simulink model "Reshape_TestGen24"  (R2017b)
settings: Solver=FixedStepDiscrete  StartTime=0.0  StopTime=10.0  RelTol=1e-3
undefined symbols (not defined in the file): Block_TestLib, enable
settings Model: Creator=ktrinh  LastModifiedBy=ktrinh
settings DebuggingCC: ParameterOverflowMsg=none

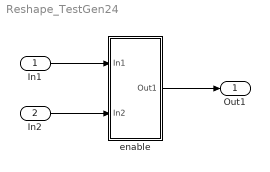
== system Reshape_TestGen24 ==
  In1 : Inport
  In2 : Inport  Port=2
  enable : Subsystem  AncestorBlock=Block_TestLib/enable
  Out1 : Outport
  wires:
  In1/1 -> enable/1(In1)
  In2/1 -> enable/2(In2)
  enable/1(Out1) -> Out1/1

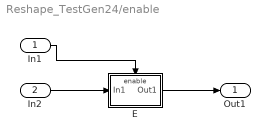
== system Reshape_TestGen24/enable ==
  In1 : Inport  OutDataTypeStr=boolean
  In2 : Inport  Port=2
  E : Subsystem  TreatAsAtomicUnit=on
  Out1 : Outport
  wires:
  In1/1 -> E/Enable
  In2/1 -> E/1(In1)
  E/1(Out1) -> Out1/1

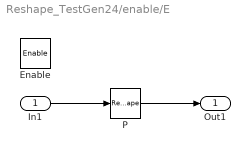
== system Reshape_TestGen24/enable/E ==
  In1 : Inport  OutDataTypeStr=int16  PortDimensions=[1,2]
  Enable : EnablePort
  P : Reshape  OutputDimensionality=Customize  OutputDimensions=[1,2]
  Out1 : Outport
  wires:
  In1/1 -> P/1
  P/1 -> Out1/1
